simulink model "Transfer_Function_Demo"  (R2022a)
settings: Solver=VariableStepAuto  StartTime=0.0  StopTime=10  RelTol=1e-3
values from neighbouring files (symbols this model uses):
  G_den = [m c k]    [Transfer_Function_Practice.m]
  G_num = [1]    [Transfer_Function_Practice.m]
settings Model: Creator=fades  LastModifiedBy=fades

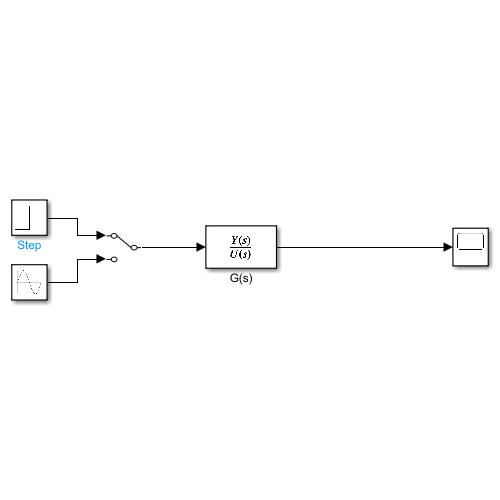
[thumbnail: Simulink's stored preview of the top-level diagram]
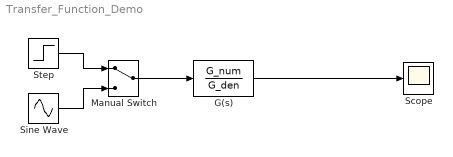
== system Transfer_Function_Demo ==
  G(s) : TransferFcn  Numerator=G_num  Denominator=G_den
  Manual Switch : ManualSwitch
  Scope : Scope
  Sine Wave : Sin  Amplitude=5  Frequency=2  SampleTime=0
  Step : Step  SampleTime=0
  wires:
  G(s)/1 -> Scope/1
  Step/1 -> Manual Switch/1
  Sine Wave/1 -> Manual Switch/2
  Manual Switch/1 -> G(s)/1
